simulink model "Racing_2019"  (R2017a)
settings: Solver=FixedStepDiscrete  StartTime=0.0  StopTime=Inf  FixedStep=1e-3  RelTol=1e-3  EnableMultiTasking=on
PostLoadFcn:
  | , if any(exist('dsrtsu_mdlpostloadfcn', 'file') == [2, 3, 6]), try dsrtsu_mdlpostloadfcn('Execute', bdroot); catch fprintf('Error in PostLoadFcn (dsrtsu_mdlpostloadfcn) for model "%s":\n %s\n', bdroot, lasterr); end, end,
undefined symbols (not defined in the file): Accu_Fans_Enable, Accu_Fans_ON, Accu_Fans_PWM, APPS_Bypass, APPS_Value, AUX_Error_Time, Batt_Temp_High_Threshold, Batt_Temp_Low_Threshold, BMS_Error_Time, BMS_Reset, BMS_Reset_Enable, BMS_Status_Bypass, Brake_Plausibility_Threshold, Brake_Threshold, Brakelight_Test, Braking_Torque, BSPD_State_Bypass, Buzzer, Buzzer_Silent, Buzzer_Test, Calibrate, CAN_Rx_FMEA_Enable, CAN_Status_FMEA_Enable, CAN_Tx_FMEA_Enable, Car_Reset, Car_Reset_Enable, Dash_Fan_PWM, DiscIntNeverNeededParam, DRS_Enable, DRS_PWM_OFF, DRS_PWM_ON, ED_Enable, ED_On, Eject_USB, Enable_Kill, Enable_LED_Test, Fans_Left_Enable, Fans_Left_ON, Fans_Left_PWM, Fans_Right_Enable, Fans_Right_ON, Fans_Right_PWM, I_MAX, IGBT_Temp_High_Threshold, IGBT_Temp_Low_Threshold, Inverter_CAN_Tx_Enable, Inverter_Frequency, KW_Max_Regen_Reset, KW_Max_Reset, LV_DCDC_Temp_High_Threshold, LV_DCDC_Temp_Low_Threshold, magnitude, Plausibility_Bypass, Power_Limiter_Killswitch, Power_Target_kW, Pump_Left_Enable, Pump_Left_ON, Pump_Right_Enable, Pump_Right_ON, Pump_Signal_Left ... (+13)
libraries: rtiusbflightreclib x206, simulink x153, rtican x52, powerlib_meascontrol x47, simulink_extras x17, rti1401lib_adc_type4 x6, rti1401lib_dio_type4 x3, rti1401lib_II_base x1
(part 19 of 23)

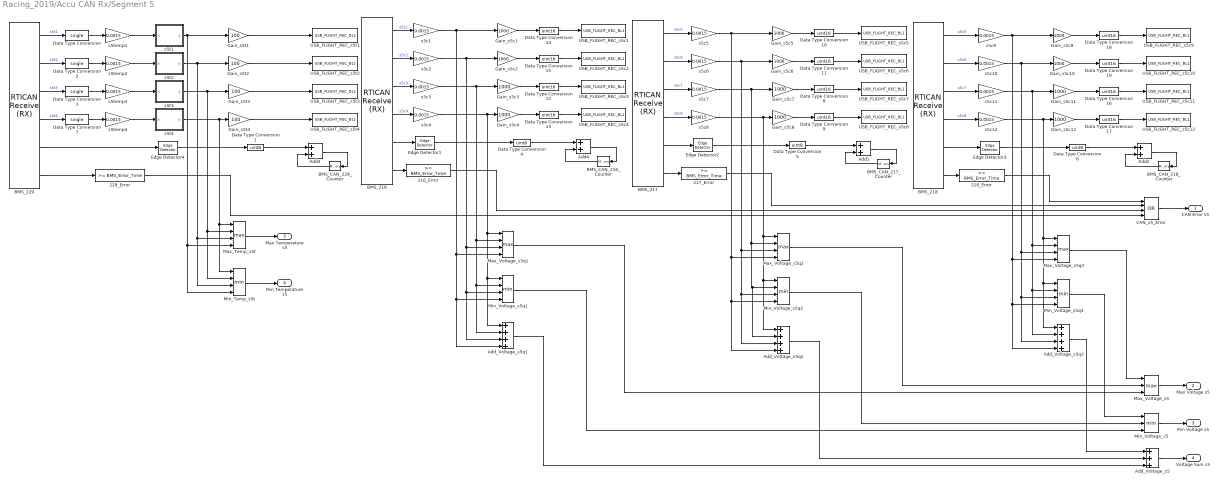
== system Racing_2019/Accu CAN Rx/Segment 5 ==
  216_Error : simulink/Logic and Bit Operations/Compare To Constant  relop=>=  const=BMS_Error_Time  OutDataTypeStr=boolean
  217_Error : simulink/Logic and Bit Operations/Compare To Constant  relop=>=  const=BMS_Error_Time  OutDataTypeStr=boolean
  218_Error : simulink/Logic and Bit Operations/Compare To Constant  relop=>=  const=BMS_Error_Time  OutDataTypeStr=boolean
  229_Error : simulink/Logic and Bit Operations/Compare To Constant  relop=>=  const=BMS_Error_Time  OutDataTypeStr=boolean
  Add{1..4} (4 alike) : Sum
  Add_Voltage_s5 : Sum  Inputs=+++
  Add_Voltage_s5q1 : Sum  Inputs=++++
  Add_Voltage_s5q2 : Sum  Inputs=++++
  Add_Voltage_s5q3 : Sum  Inputs=++++
  BMS_216 : rtican/RTICAN Receive (RX)   Reserved1=[]  Reserved2=[]  Reserved3=[]  Reserved4=[]  SfcnMessage=[]  Msg_Struct=[]  BoardTypeNo=[]  BoardNo=[]  ChannelNo=[]  Parameters=[]  DialogFcn=[]  UnitName=[]  Revision=[]  UnitValues=[]  DSProperties=struct('RTI',struct('Version',uint32(5),'BlockType',struct('isSLSource',uint8(1),'isSLSink',uint8(1),'isHWSource',uint8(0),'isHWSink',uint8(0),'isSetup',uint8(0),'isInline',uint8(1),'isNonInline',uint8(0),'isInterrupt',uint8(0),'isChannelwise',uint8(0)),'IOBoardType','RTICAN','UnitType','MESSAGE','Identifier','RX','DialogType','MSVC','BlockSet','RTICAN','SlaveProcessor','CAN'))  RTIBlockInterface=struct('OutputPortsWidth',int32([1 1 1 1 1 1]),'OutputPortsActive',[1 1 1 1 1 1],'OutputPortsName',{{'s5c1','s5c2','s5c3','s5c4',['RX status'],['RX delta time']}},'OutputPortsDataType',{{'SS_DOUBLE','SS_DOUBLE','SS_DOUBLE','SS_DOUBLE','SS_DOUBLE','SS_DOUBLE'}},'OutputPortsLabel',{{'s5c1','s5c2','s5c3','s5c4','',''}},'OutputPortsLabelMode','ON','InputPortsWidth',int32(0),'InputPortsActive',0,'DialogFcn','rtican_message_interface_gui','BlockDisplay',{{'','center'}},'IconTransparency','on','ParameterTunableNames',{{}},'InitLevel',3,'BlockName',struct('Token',{{'CAN_TYPE','_RX_M','_C'}},'BlockParam',{{'BoardTypeNo','BoardNo','ChannelNo'}}),'SampleTime',{{0.2}},'TriggerPort',{{'none'}},'EnablePort',{{'none'}})  RTIBlockParameters=struct('BoardTypeNo',{{1,'OFF',[]}},'BoardNo',{{2,'ON',[1 16]}},'ChannelNo',{{1,'ON',[1 2]}},'Parameters',{{struct('DataFileSupport',struct('DataFileSelectedMaster',0,'DataFileSelectedLocal',0,'DataFileName',['<no datafile support>|'],'DataFileDate','','SelectedFile',['<no file selected>']),'Options',struct('StatusSelected',1,'TimeSelected',0,'DeltaTimeSelected',1,'BytePortSelected',0,'MessageLengthSelected',0,'TriggerPort',struct('Selected',0,'TriggerType',0),'UserCoding',struct('Selected',0,'InterfaceFile','UserDecodingFile','FcnName','UserDecodeFcn','InportSelected',0,'InportWidth',1,'OutportSelected',0,'OutportWidth',1),'EnablePortSelected',0,'SignalOnPortnameSelected',1,'UseRXService',0),'Message',struct('MsgOnBlocknameSelected',0,'MsgName','BMS_s5q1','MsgIdFormat',0,'MsgId',216,'MsgLength',8,'NumSignals',4,'SampleTime',0.2,'Signal',struct('SgnName',{'s5c1','s5c2','s5c3','s5c4'},'SgnStartBit',{0,16,32,48},'SgnLength',{16,16,16,16},'SgnType',{0,0,0,0},'ModeValue',{-1,-1,-1,-1},'DataType',{0,0,0,0},'ByteLayout',{1,1,1,1},'Factor',{1,1,1,1},'Offset',{0,0,0,0},'SgnComment',{{''},{''},{''},{''}},'SgnUnit',{'','','',''},'Min',{0,0,0,0},'Max',{255,255,255,255},'SLDataType',{'SS_DOUBLE','SS_DOUBLE','SS_DOUBLE','SS_DOUBLE'}),'MsgIdNumFormat',0,'MsgComment',{{''}}),'Version',1.2,'general',struct('isFromLib',0)),'OFF',[]}},'GroupId',{{struct('Group',{{'RTICAN'}},'No',3,'Behavior',{{'NAMECHANGE'}},'BlockType',{{'SINK'}},'NameChangeFlag',0),'OFF',[]}},'SFcnRTICANMessage',{{struct('MsgType','RX','SFcnPortType','Scalar','MsgName','BMS_s5q1','MsgIdFormat','STD','MsgId',216,'MsgLength',8,'NumSignals',4,'SampleTime',0.2,'Signal',struct('SgnName',{'s5c1','s5c2','s5c3','s5c4'},'SgnStartBit',{0,16,32,48},'SgnLength',{16,16,16,16},'SgnType',{'standard','standard','standard','standard'},'ModeValue',{-1,-1,-1,-1},'DataType',{['unsigned int'],['unsigned int'],['unsigned int'],['unsigned int']},'ByteLayout',{['big endian'],['big endian'],['big endian'],['big endian']},'Factor',{1,1,1,1},'Offset',{0,0,0,0},'SLDataType',{'SS_DOUBLE','SS_DOUBLE','SS_DOUBLE','SS_DOUBLE'}),'StatusSelected','yes','TimeSelected','no','DeltaTimeSelected','yes','BytePortSelected','no','MessageLengthSelected','no','TriggerPort',struct('Selected','no','TriggerType',0),'UserCoding',struct('Selected','no','InterfaceFile','UserDecodingFile','FcnName','UserDecodeFcn','InportSelected','no','InportWidth',1,'OutportSelected','no','OutportWidth',1),'EnablePortSelected','no','UseRXService','no','BoardType','DS1','BoardNo',2,'ControllerNo',1),'OFF',[]}},'TLCFileName',{{'rtican_rx_message','OFF',[]}})  RTISFcnParameters=struct('SFcnRTICANMessage','struct','TLCFileName','char')  RTIBlockParaDefault=struct('BoardTypeNo',4302,'BoardNo',1,'ChannelNo',1,'Parameters',struct('DataFileSupport',struct('DataFileSelectedMaster',0,'DataFileSelectedLocal',0,'DataFileName','','DataFileDate','','SelectedFile',['<no file selected>']),'Options',struct('StatusSelected',1,'TimeSelected',1,'DeltaTimeSelected',1,'BytePortSelected',0,'MessageLengthSelected',0,'TriggerPort',struct('Selected',0,'TriggerType','rising'),'UserCoding',struct('Selected',0,'InterfaceFile','UserDecodingFile','FcnName','UserDecodeFcn','InportSelected',0,'InportWidth',1,'OutportSelected',0,'OutportWidth',1),'EnablePortSelected',0,'SignalOnPortnameSelected',1,'UseRXService',0),'Message',struct('MsgOnBlocknameSelected',0,'MsgName',['RX Message'],'MsgIdFormat',0,'MsgId',100,'MsgLength',8,'NumSignals',1,'SampleTime',-1,'Signal',struct('SgnName',['RX signal'],'SgnStartBit',0,'SgnLength',8,'SgnType',0,'ModeValue',-1,'DataType',0,'SLDataType','SS_DOUBLE','ByteLayout',0,'Factor',1,'Offset',0,'Min',0,'Max',255,'SgnComment',{{}},'SgnUnit',''),'MsgIdNumFormat',0,'MsgComment',{{''}}),'Version',1.2,'general',struct('isFromLib',1)),'GroupId',struct('Group',{{'RTICAN'}},'No',1,'Behavior',{{'NAMECHANGE'}},'BlockType',{{'SINK'}},'NameChangeFlag',0),'SFcnRTICANMessage',struct('MsgType','RX','MsgName',['RX Message'],'MsgIdFormat','STD','MsgId',100,'MsgLength',8,'NumSignals',1,'SampleTime',-1,'Signal',struct('SgnName',['RX signal'],'SgnStartBit',0,'SgnLength',8,'SgnType','standard','ModeValue',-1,'DataType',['unsigned int'],'ByteLayout',['little endian'],'SLDataType','SS_DOUBLE','Factor',1,'Offset',0),'StatusSelected','yes','TimeSelected','yes','DeltaTimeSelected','yes','BytePortSelected','no','MessageLengthSelected','no','EnablePortSelected','no','UserCoding',struct('Selected','no','InterfaceFile','UserDecodingFile','FcnName','UserDecodeFcn','InportSelected','no','InportWidth',1,'OutportSelected','no','OutportWidth',1),'TriggerPort',struct('Selected','no','TriggerType','rising'),'UseRXService','no','BoardType','DS4302','BoardNo',1,'ControllerNo',1,'SFcnPortType','Scalar'),'TLCFileName','rtican_rx_message')
      settings: AttributesFormatString=Group Id: RTICAN3\n  SourceProductName=dSPACE RTI CAN Blockset
  BMS_217 : rtican/RTICAN Receive (RX)   Reserved1=[]  Reserved2=[]  Reserved3=[]  Reserved4=[]  SfcnMessage=[]  Msg_Struct=[]  BoardTypeNo=[]  BoardNo=[]  ChannelNo=[]  Parameters=[]  DialogFcn=[]  UnitName=[]  Revision=[]  UnitValues=[]  DSProperties=struct('RTI',struct('Version',uint32(5),'BlockType',struct('isSLSource',uint8(1),'isSLSink',uint8(1),'isHWSource',uint8(0),'isHWSink',uint8(0),'isSetup',uint8(0),'isInline',uint8(1),'isNonInline',uint8(0),'isInterrupt',uint8(0),'isChannelwise',uint8(0)),'IOBoardType','RTICAN','UnitType','MESSAGE','Identifier','RX','DialogType','MSVC','BlockSet','RTICAN','SlaveProcessor','CAN'))  RTIBlockInterface=struct('OutputPortsWidth',int32([1 1 1 1 1 1]),'OutputPortsActive',[1 1 1 1 1 1],'OutputPortsName',{{'s5c5','s5c6','s5c7','s5c8',['RX status'],['RX delta time']}},'OutputPortsDataType',{{'SS_DOUBLE','SS_DOUBLE','SS_DOUBLE','SS_DOUBLE','SS_DOUBLE','SS_DOUBLE'}},'OutputPortsLabel',{{'s5c5','s5c6','s5c7','s5c8','',''}},'OutputPortsLabelMode','ON','InputPortsWidth',int32(0),'InputPortsActive',0,'DialogFcn','rtican_message_interface_gui','BlockDisplay',{{'','center'}},'IconTransparency','on','ParameterTunableNames',{{}},'InitLevel',3,'BlockName',struct('Token',{{'CAN_TYPE','_RX_M','_C'}},'BlockParam',{{'BoardTypeNo','BoardNo','ChannelNo'}}),'SampleTime',{{0.2}},'TriggerPort',{{'none'}},'EnablePort',{{'none'}})  RTIBlockParameters=struct('BoardTypeNo',{{1,'OFF',[]}},'BoardNo',{{2,'ON',[1 16]}},'ChannelNo',{{1,'ON',[1 2]}},'Parameters',{{struct('DataFileSupport',struct('DataFileSelectedMaster',0,'DataFileSelectedLocal',0,'DataFileName',['<no datafile support>|'],'DataFileDate','','SelectedFile',['<no file selected>']),'Options',struct('StatusSelected',1,'TimeSelected',0,'DeltaTimeSelected',1,'BytePortSelected',0,'MessageLengthSelected',0,'TriggerPort',struct('Selected',0,'TriggerType',0),'UserCoding',struct('Selected',0,'InterfaceFile','UserDecodingFile','FcnName','UserDecodeFcn','InportSelected',0,'InportWidth',1,'OutportSelected',0,'OutportWidth',1),'EnablePortSelected',0,'SignalOnPortnameSelected',1,'UseRXService',0),'Message',struct('MsgOnBlocknameSelected',0,'MsgName','BMS_s5q2','MsgIdFormat',0,'MsgId',217,'MsgLength',8,'NumSignals',4,'SampleTime',0.2,'Signal',struct('SgnName',{'s5c5','s5c6','s5c7','s5c8'},'SgnStartBit',{0,16,32,48},'SgnLength',{16,16,16,16},'SgnType',{0,0,0,0},'ModeValue',{-1,-1,-1,-1},'DataType',{0,0,0,0},'ByteLayout',{1,1,1,1},'Factor',{1,1,1,1},'Offset',{0,0,0,0},'SgnComment',{{''},{''},{''},{''}},'SgnUnit',{'','','',''},'Min',{0,0,0,0},'Max',{255,255,255,255},'SLDataType',{'SS_DOUBLE','SS_DOUBLE','SS_DOUBLE','SS_DOUBLE'}),'MsgIdNumFormat',0,'MsgComment',{{''}}),'Version',1.2,'general',struct('isFromLib',0)),'OFF',[]}},'GroupId',{{struct('Group',{{'RTICAN'}},'No',3,'Behavior',{{'NAMECHANGE'}},'BlockType',{{'SINK'}},'NameChangeFlag',0),'OFF',[]}},'SFcnRTICANMessage',{{struct('MsgType','RX','SFcnPortType','Scalar','MsgName','BMS_s5q2','MsgIdFormat','STD','MsgId',217,'MsgLength',8,'NumSignals',4,'SampleTime',0.2,'Signal',struct('SgnName',{'s5c5','s5c6','s5c7','s5c8'},'SgnStartBit',{0,16,32,48},'SgnLength',{16,16,16,16},'SgnType',{'standard','standard','standard','standard'},'ModeValue',{-1,-1,-1,-1},'DataType',{['unsigned int'],['unsigned int'],['unsigned int'],['unsigned int']},'ByteLayout',{['big endian'],['big endian'],['big endian'],['big endian']},'Factor',{1,1,1,1},'Offset',{0,0,0,0},'SLDataType',{'SS_DOUBLE','SS_DOUBLE','SS_DOUBLE','SS_DOUBLE'}),'StatusSelected','yes','TimeSelected','no','DeltaTimeSelected','yes','BytePortSelected','no','MessageLengthSelected','no','TriggerPort',struct('Selected','no','TriggerType',0),'UserCoding',struct('Selected','no','InterfaceFile','UserDecodingFile','FcnName','UserDecodeFcn','InportSelected','no','InportWidth',1,'OutportSelected','no','OutportWidth',1),'EnablePortSelected','no','UseRXService','no','BoardType','DS1','BoardNo',2,'ControllerNo',1),'OFF',[]}},'TLCFileName',{{'rtican_rx_message','OFF',[]}})  RTISFcnParameters=struct('SFcnRTICANMessage','struct','TLCFileName','char')  RTIBlockParaDefault=struct('BoardTypeNo',4302,'BoardNo',1,'ChannelNo',1,'Parameters',struct('DataFileSupport',struct('DataFileSelectedMaster',0,'DataFileSelectedLocal',0,'DataFileName','','DataFileDate','','SelectedFile',['<no file selected>']),'Options',struct('StatusSelected',1,'TimeSelected',1,'DeltaTimeSelected',1,'BytePortSelected',0,'MessageLengthSelected',0,'TriggerPort',struct('Selected',0,'TriggerType','rising'),'UserCoding',struct('Selected',0,'InterfaceFile','UserDecodingFile','FcnName','UserDecodeFcn','InportSelected',0,'InportWidth',1,'OutportSelected',0,'OutportWidth',1),'EnablePortSelected',0,'SignalOnPortnameSelected',1,'UseRXService',0),'Message',struct('MsgOnBlocknameSelected',0,'MsgName',['RX Message'],'MsgIdFormat',0,'MsgId',100,'MsgLength',8,'NumSignals',1,'SampleTime',-1,'Signal',struct('SgnName',['RX signal'],'SgnStartBit',0,'SgnLength',8,'SgnType',0,'ModeValue',-1,'DataType',0,'SLDataType','SS_DOUBLE','ByteLayout',0,'Factor',1,'Offset',0,'Min',0,'Max',255,'SgnComment',{{}},'SgnUnit',''),'MsgIdNumFormat',0,'MsgComment',{{''}}),'Version',1.2,'general',struct('isFromLib',1)),'GroupId',struct('Group',{{'RTICAN'}},'No',1,'Behavior',{{'NAMECHANGE'}},'BlockType',{{'SINK'}},'NameChangeFlag',0),'SFcnRTICANMessage',struct('MsgType','RX','MsgName',['RX Message'],'MsgIdFormat','STD','MsgId',100,'MsgLength',8,'NumSignals',1,'SampleTime',-1,'Signal',struct('SgnName',['RX signal'],'SgnStartBit',0,'SgnLength',8,'SgnType','standard','ModeValue',-1,'DataType',['unsigned int'],'ByteLayout',['little endian'],'SLDataType','SS_DOUBLE','Factor',1,'Offset',0),'StatusSelected','yes','TimeSelected','yes','DeltaTimeSelected','yes','BytePortSelected','no','MessageLengthSelected','no','EnablePortSelected','no','UserCoding',struct('Selected','no','InterfaceFile','UserDecodingFile','FcnName','UserDecodeFcn','InportSelected','no','InportWidth',1,'OutportSelected','no','OutportWidth',1),'TriggerPort',struct('Selected','no','TriggerType','rising'),'UseRXService','no','BoardType','DS4302','BoardNo',1,'ControllerNo',1,'SFcnPortType','Scalar'),'TLCFileName','rtican_rx_message')
      settings: AttributesFormatString=Group Id: RTICAN3\n  SourceProductName=dSPACE RTI CAN Blockset
  BMS_218 : rtican/RTICAN Receive (RX)   Reserved1=[]  Reserved2=[]  Reserved3=[]  Reserved4=[]  SfcnMessage=[]  Msg_Struct=[]  BoardTypeNo=[]  BoardNo=[]  ChannelNo=[]  Parameters=[]  DialogFcn=[]  UnitName=[]  Revision=[]  UnitValues=[]  DSProperties=struct('RTI',struct('Version',uint32(5),'BlockType',struct('isSLSource',uint8(1),'isSLSink',uint8(1),'isHWSource',uint8(0),'isHWSink',uint8(0),'isSetup',uint8(0),'isInline',uint8(1),'isNonInline',uint8(0),'isInterrupt',uint8(0),'isChannelwise',uint8(0)),'IOBoardType','RTICAN','UnitType','MESSAGE','Identifier','RX','DialogType','MSVC','BlockSet','RTICAN','SlaveProcessor','CAN'))  RTIBlockInterface=struct('OutputPortsWidth',int32([1 1 1 1 1 1]),'OutputPortsActive',[1 1 1 1 1 1],'OutputPortsName',{{'s5c5','s5c6','s5c7','s5c8',['RX status'],['RX delta time']}},'OutputPortsDataType',{{'SS_DOUBLE','SS_DOUBLE','SS_DOUBLE','SS_DOUBLE','SS_DOUBLE','SS_DOUBLE'}},'OutputPortsLabel',{{'s5c5','s5c6','s5c7','s5c8','',''}},'OutputPortsLabelMode','ON','InputPortsWidth',int32(0),'InputPortsActive',0,'DialogFcn','rtican_message_interface_gui','BlockDisplay',{{'','center'}},'IconTransparency','on','ParameterTunableNames',{{}},'InitLevel',3,'BlockName',struct('Token',{{'CAN_TYPE','_RX_M','_C'}},'BlockParam',{{'BoardTypeNo','BoardNo','ChannelNo'}}),'SampleTime',{{0.2}},'TriggerPort',{{'none'}},'EnablePort',{{'none'}})  RTIBlockParameters=struct('BoardTypeNo',{{1,'OFF',[]}},'BoardNo',{{2,'ON',[1 16]}},'ChannelNo',{{1,'ON',[1 2]}},'Parameters',{{struct('DataFileSupport',struct('DataFileSelectedMaster',0,'DataFileSelectedLocal',0,'DataFileName',['<no datafile support>|'],'DataFileDate','','SelectedFile',['<no file selected>']),'Options',struct('StatusSelected',1,'TimeSelected',0,'DeltaTimeSelected',1,'BytePortSelected',0,'MessageLengthSelected',0,'TriggerPort',struct('Selected',0,'TriggerType',0),'UserCoding',struct('Selected',0,'InterfaceFile','UserDecodingFile','FcnName','UserDecodeFcn','InportSelected',0,'InportWidth',1,'OutportSelected',0,'OutportWidth',1),'EnablePortSelected',0,'SignalOnPortnameSelected',1,'UseRXService',0),'Message',struct('MsgOnBlocknameSelected',0,'MsgName','BMS_s5q3','MsgIdFormat',0,'MsgId',218,'MsgLength',8,'NumSignals',4,'SampleTime',0.2,'Signal',struct('SgnName',{'s5c5','s5c6','s5c7','s5c8'},'SgnStartBit',{0,16,32,48},'SgnLength',{16,16,16,16},'SgnType',{0,0,0,0},'ModeValue',{-1,-1,-1,-1},'DataType',{0,0,0,0},'ByteLayout',{1,1,1,1},'Factor',{1,1,1,1},'Offset',{0,0,0,0},'SgnComment',{{''},{''},{''},{''}},'SgnUnit',{'','','',''},'Min',{0,0,0,0},'Max',{255,255,255,255},'SLDataType',{'SS_DOUBLE','SS_DOUBLE','SS_DOUBLE','SS_DOUBLE'}),'MsgIdNumFormat',0,'MsgComment',{{''}}),'Version',1.2,'general',struct('isFromLib',0)),'OFF',[]}},'GroupId',{{struct('Group',{{'RTICAN'}},'No',3,'Behavior',{{'NAMECHANGE'}},'BlockType',{{'SINK'}},'NameChangeFlag',0),'OFF',[]}},'SFcnRTICANMessage',{{struct('MsgType','RX','SFcnPortType','Scalar','MsgName','BMS_s5q3','MsgIdFormat','STD','MsgId',218,'MsgLength',8,'NumSignals',4,'SampleTime',0.2,'Signal',struct('SgnName',{'s5c5','s5c6','s5c7','s5c8'},'SgnStartBit',{0,16,32,48},'SgnLength',{16,16,16,16},'SgnType',{'standard','standard','standard','standard'},'ModeValue',{-1,-1,-1,-1},'DataType',{['unsigned int'],['unsigned int'],['unsigned int'],['unsigned int']},'ByteLayout',{['big endian'],['big endian'],['big endian'],['big endian']},'Factor',{1,1,1,1},'Offset',{0,0,0,0},'SLDataType',{'SS_DOUBLE','SS_DOUBLE','SS_DOUBLE','SS_DOUBLE'}),'StatusSelected','yes','TimeSelected','no','DeltaTimeSelected','yes','BytePortSelected','no','MessageLengthSelected','no','TriggerPort',struct('Selected','no','TriggerType',0),'UserCoding',struct('Selected','no','InterfaceFile','UserDecodingFile','FcnName','UserDecodeFcn','InportSelected','no','InportWidth',1,'OutportSelected','no','OutportWidth',1),'EnablePortSelected','no','UseRXService','no','BoardType','DS1','BoardNo',2,'ControllerNo',1),'OFF',[]}},'TLCFileName',{{'rtican_rx_message','OFF',[]}})  RTISFcnParameters=struct('SFcnRTICANMessage','struct','TLCFileName','char')  RTIBlockParaDefault=struct('BoardTypeNo',4302,'BoardNo',1,'ChannelNo',1,'Parameters',struct('DataFileSupport',struct('DataFileSelectedMaster',0,'DataFileSelectedLocal',0,'DataFileName','','DataFileDate','','SelectedFile',['<no file selected>']),'Options',struct('StatusSelected',1,'TimeSelected',1,'DeltaTimeSelected',1,'BytePortSelected',0,'MessageLengthSelected',0,'TriggerPort',struct('Selected',0,'TriggerType','rising'),'UserCoding',struct('Selected',0,'InterfaceFile','UserDecodingFile','FcnName','UserDecodeFcn','InportSelected',0,'InportWidth',1,'OutportSelected',0,'OutportWidth',1),'EnablePortSelected',0,'SignalOnPortnameSelected',1,'UseRXService',0),'Message',struct('MsgOnBlocknameSelected',0,'MsgName',['RX Message'],'MsgIdFormat',0,'MsgId',100,'MsgLength',8,'NumSignals',1,'SampleTime',-1,'Signal',struct('SgnName',['RX signal'],'SgnStartBit',0,'SgnLength',8,'SgnType',0,'ModeValue',-1,'DataType',0,'SLDataType','SS_DOUBLE','ByteLayout',0,'Factor',1,'Offset',0,'Min',0,'Max',255,'SgnComment',{{}},'SgnUnit',''),'MsgIdNumFormat',0,'MsgComment',{{''}}),'Version',1.2,'general',struct('isFromLib',1)),'GroupId',struct('Group',{{'RTICAN'}},'No',1,'Behavior',{{'NAMECHANGE'}},'BlockType',{{'SINK'}},'NameChangeFlag',0),'SFcnRTICANMessage',struct('MsgType','RX','MsgName',['RX Message'],'MsgIdFormat','STD','MsgId',100,'MsgLength',8,'NumSignals',1,'SampleTime',-1,'Signal',struct('SgnName',['RX signal'],'SgnStartBit',0,'SgnLength',8,'SgnType','standard','ModeValue',-1,'DataType',['unsigned int'],'ByteLayout',['little endian'],'SLDataType','SS_DOUBLE','Factor',1,'Offset',0),'StatusSelected','yes','TimeSelected','yes','DeltaTimeSelected','yes','BytePortSelected','no','MessageLengthSelected','no','EnablePortSelected','no','UserCoding',struct('Selected','no','InterfaceFile','UserDecodingFile','FcnName','UserDecodeFcn','InportSelected','no','InportWidth',1,'OutportSelected','no','OutportWidth',1),'TriggerPort',struct('Selected','no','TriggerType','rising'),'UseRXService','no','BoardType','DS4302','BoardNo',1,'ControllerNo',1,'SFcnPortType','Scalar'),'TLCFileName','rtican_rx_message')
      settings: AttributesFormatString=Group Id: RTICAN3\n  SourceProductName=dSPACE RTI CAN Blockset
  BMS_229 : rtican/RTICAN Receive (RX)   Reserved1=[]  Reserved2=[]  Reserved3=[]  Reserved4=[]  SfcnMessage=[]  Msg_Struct=[]  BoardTypeNo=[]  BoardNo=[]  ChannelNo=[]  Parameters=[]  DialogFcn=[]  UnitName=[]  Revision=[]  UnitValues=[]  DSProperties=struct('RTI',struct('Version',uint32(5),'BlockType',struct('isSLSource',uint8(1),'isSLSink',uint8(1),'isHWSource',uint8(0),'isHWSink',uint8(0),'isSetup',uint8(0),'isInline',uint8(1),'isNonInline',uint8(0),'isInterrupt',uint8(0),'isChannelwise',uint8(0)),'IOBoardType','RTICAN','UnitType','MESSAGE','Identifier','RX','DialogType','MSVC','BlockSet','RTICAN','SlaveProcessor','CAN'))  RTIBlockInterface=struct('OutputPortsWidth',int32([1 1 1 1 1 1]),'OutputPortsActive',[1 1 1 1 1 1],'OutputPortsName',{{'s5t1','s5t2','s5t3','s5t4',['RX status'],['RX delta time']}},'OutputPortsDataType',{{'SS_DOUBLE','SS_DOUBLE','SS_DOUBLE','SS_DOUBLE','SS_DOUBLE','SS_DOUBLE'}},'OutputPortsLabel',{{'s5t1','s5t2','s5t3','s5t4','',''}},'OutputPortsLabelMode','ON','InputPortsWidth',int32(0),'InputPortsActive',0,'DialogFcn','rtican_message_interface_gui','BlockDisplay',{{'','center'}},'IconTransparency','on','ParameterTunableNames',{{}},'InitLevel',3,'BlockName',struct('Token',{{'CAN_TYPE','_RX_M','_C'}},'BlockParam',{{'BoardTypeNo','BoardNo','ChannelNo'}}),'SampleTime',{{0.2}},'TriggerPort',{{'none'}},'EnablePort',{{'none'}})  RTIBlockParameters=struct('BoardTypeNo',{{1,'OFF',[]}},'BoardNo',{{2,'ON',[1 16]}},'ChannelNo',{{1,'ON',[1 2]}},'Parameters',{{struct('DataFileSupport',struct('DataFileSelectedMaster',0,'DataFileSelectedLocal',0,'DataFileName',['<no datafile support>|'],'DataFileDate','','SelectedFile',['<no file selected>']),'Options',struct('StatusSelected',1,'TimeSelected',0,'DeltaTimeSelected',1,'BytePortSelected',0,'MessageLengthSelected',0,'TriggerPort',struct('Selected',0,'TriggerType',0),'UserCoding',struct('Selected',0,'InterfaceFile','UserDecodingFile','FcnName','UserDecodeFcn','InportSelected',0,'InportWidth',1,'OutportSelected',0,'OutportWidth',1),'EnablePortSelected',0,'SignalOnPortnameSelected',1,'UseRXService',0),'Message',struct('MsgOnBlocknameSelected',0,'MsgName','BMS_s5t','MsgIdFormat',0,'MsgId',229,'MsgLength',8,'NumSignals',4,'SampleTime',0.2,'Signal',struct('SgnName',{'s5t1','s5t2','s5t3','s5t4'},'SgnStartBit',{0,16,32,48},'SgnLength',{16,16,16,16},'SgnType',{0,0,0,0},'ModeValue',{-1,-1,-1,-1},'DataType',{0,0,0,0},'ByteLayout',{1,1,1,1},'Factor',{1,1,1,1},'Offset',{0,0,0,0},'SgnComment',{{''},{''},{''},{''}},'SgnUnit',{'','','',''},'Min',{0,0,0,0},'Max',{255,255,255,255},'SLDataType',{'SS_DOUBLE','SS_DOUBLE','SS_DOUBLE','SS_DOUBLE'}),'MsgIdNumFormat',0,'MsgComment',{{''}}),'Version',1.2,'general',struct('isFromLib',0)),'OFF',[]}},'GroupId',{{struct('Group',{{'RTICAN'}},'No',3,'Behavior',{{'NAMECHANGE'}},'BlockType',{{'SINK'}},'NameChangeFlag',0),'OFF',[]}},'SFcnRTICANMessage',{{struct('MsgType','RX','SFcnPortType','Scalar','MsgName','BMS_s5t','MsgIdFormat','STD','MsgId',229,'MsgLength',8,'NumSignals',4,'SampleTime',0.2,'Signal',struct('SgnName',{'s5t1','s5t2','s5t3','s5t4'},'SgnStartBit',{0,16,32,48},'SgnLength',{16,16,16,16},'SgnType',{'standard','standard','standard','standard'},'ModeValue',{-1,-1,-1,-1},'DataType',{['unsigned int'],['unsigned int'],['unsigned int'],['unsigned int']},'ByteLayout',{['big endian'],['big endian'],['big endian'],['big endian']},'Factor',{1,1,1,1},'Offset',{0,0,0,0},'SLDataType',{'SS_DOUBLE','SS_DOUBLE','SS_DOUBLE','SS_DOUBLE'}),'StatusSelected','yes','TimeSelected','no','DeltaTimeSelected','yes','BytePortSelected','no','MessageLengthSelected','no','TriggerPort',struct('Selected','no','TriggerType',0),'UserCoding',struct('Selected','no','InterfaceFile','UserDecodingFile','FcnName','UserDecodeFcn','InportSelected','no','InportWidth',1,'OutportSelected','no','OutportWidth',1),'EnablePortSelected','no','UseRXService','no','BoardType','DS1','BoardNo',2,'ControllerNo',1),'OFF',[]}},'TLCFileName',{{'rtican_rx_message','OFF',[]}})  RTISFcnParameters=struct('SFcnRTICANMessage','struct','TLCFileName','char')  RTIBlockParaDefault=struct('BoardTypeNo',4302,'BoardNo',1,'ChannelNo',1,'Parameters',struct('DataFileSupport',struct('DataFileSelectedMaster',0,'DataFileSelectedLocal',0,'DataFileName','','DataFileDate','','SelectedFile',['<no file selected>']),'Options',struct('StatusSelected',1,'TimeSelected',1,'DeltaTimeSelected',1,'BytePortSelected',0,'MessageLengthSelected',0,'TriggerPort',struct('Selected',0,'TriggerType','rising'),'UserCoding',struct('Selected',0,'InterfaceFile','UserDecodingFile','FcnName','UserDecodeFcn','InportSelected',0,'InportWidth',1,'OutportSelected',0,'OutportWidth',1),'EnablePortSelected',0,'SignalOnPortnameSelected',1,'UseRXService',0),'Message',struct('MsgOnBlocknameSelected',0,'MsgName',['RX Message'],'MsgIdFormat',0,'MsgId',100,'MsgLength',8,'NumSignals',1,'SampleTime',-1,'Signal',struct('SgnName',['RX signal'],'SgnStartBit',0,'SgnLength',8,'SgnType',0,'ModeValue',-1,'DataType',0,'SLDataType','SS_DOUBLE','ByteLayout',0,'Factor',1,'Offset',0,'Min',0,'Max',255,'SgnComment',{{}},'SgnUnit',''),'MsgIdNumFormat',0,'MsgComment',{{''}}),'Version',1.2,'general',struct('isFromLib',1)),'GroupId',struct('Group',{{'RTICAN'}},'No',1,'Behavior',{{'NAMECHANGE'}},'BlockType',{{'SINK'}},'NameChangeFlag',0),'SFcnRTICANMessage',struct('MsgType','RX','MsgName',['RX Message'],'MsgIdFormat','STD','MsgId',100,'MsgLength',8,'NumSignals',1,'SampleTime',-1,'Signal',struct('SgnName',['RX signal'],'SgnStartBit',0,'SgnLength',8,'SgnType','standard','ModeValue',-1,'DataType',['unsigned int'],'ByteLayout',['little endian'],'SLDataType','SS_DOUBLE','Factor',1,'Offset',0),'StatusSelected','yes','TimeSelected','yes','DeltaTimeSelected','yes','BytePortSelected','no','MessageLengthSelected','no','EnablePortSelected','no','UserCoding',struct('Selected','no','InterfaceFile','UserDecodingFile','FcnName','UserDecodeFcn','InportSelected','no','InportWidth',1,'OutportSelected','no','OutportWidth',1),'TriggerPort',struct('Selected','no','TriggerType','rising'),'UseRXService','no','BoardType','DS4302','BoardNo',1,'ControllerNo',1,'SFcnPortType','Scalar'),'TLCFileName','rtican_rx_message')
      settings: AttributesFormatString=Group Id: RTICAN3\n  SourceProductName=dSPACE RTI CAN Blockset
  BMS_CAN_216_Counter : Memory  InheritSampleTime=on
  BMS_CAN_217_Counter : Memory  InheritSampleTime=on
  BMS_CAN_218_Counter : Memory  InheritSampleTime=on
  BMS_CAN_229_Counter : Memory  InheritSampleTime=on
  CAN_s5_Error : Logic  Operator=OR  Inputs=4  AllPortsSameDT=off  OutDataTypeStr=boolean
  Data Type Conversion{,2..3,7} (4 alike) : DataTypeConversion  OutDataTypeStr=single
  Data Type Conversion{1,4..6} (4 alike) : DataTypeConversion  OutDataTypeStr=uint8
  Data Type Conversion{8..19} (12 alike) : DataTypeConversion  OutDataTypeStr=uint16
  Edge Detector{1..4} (4 alike) : powerlib_meascontrol/Logic/Edge Detector  model=Rising  ic=0  Ts=-1
      settings: SourceProductName=Simscape Power Systems  SourceProductBaseCode=PS
  Gain_s5c{1..12} (12 alike) : Gain  Gain=1000
  Gain_s5t{1..4} (4 alike) : Gain  Gain=100
  Max_Temp_s5t : MinMax  Function=max  Inputs=4
  Max_Voltage_s5 : MinMax  Function=max  Inputs=3
  Max_Voltage_s5q1 : MinMax  Function=max  Inputs=4
  Max_Voltage_s5q2 : MinMax  Function=max  Inputs=4
  Max_Voltage_s5q3 : MinMax  Function=max  Inputs=4
  Min_Temp_s5t : MinMax  Inputs=4
  Min_Voltage_s5 : MinMax  Inputs=3
  Min_Voltage_s5q1 : MinMax  Inputs=4
  Min_Voltage_s5q2 : MinMax  Inputs=4
  Min_Voltage_s5q3 : MinMax  Inputs=4
  USB_FLIGHT_REC_s5c1 : rtiusbflightreclib/USB_FLIGHT_REC_BL1  VarName=s5c1  DataType=UInt16  SampleTime=-1  TLCFileName=rtiusbflightrecwrite  Reserved1=[]  Reserved2=[]  Reserved3=[]  Reserved4=[]  DSProperties=struct('RTI',struct('Version',uint32(3),'BlockType',struct('isSLSource',uint8(0),'isSLSink',uint8(1),'isHWSource',uint8(0),'isHWSink',uint8(0),'isSetup',uint8(0),'isInline',uint8(1),'isNonInline',uint8(0),'isInterrupt',uint8(0),'isChannelwise',uint8(0)),'IOBoardType',{{'DSUSB','FLIGHTREC'}},'UnitType','FLIGHTREC','Identifier','WRITE','DialogType','SL','BlockSet','RTIUSBFLIGHTREC','SlaveProcessor','NONE'))  RTIBlockInterface=struct('InputPortsActive',1,'InputPortsWidth',int32(1),'InputPortsDataType',{{'SS_UINT16'}},'BlockDisplay',{{['Write to\nUSB Flight Recorder'],'center'}},'IconTransparency','off','InitLevel',3,'BlockName',struct('Token',{{'USB_FLIGHT_REC_BL1'}}),'MaskDescription',['Write input to the Flight Recorder. Recorded data can be referenced by the specified variable.'],'SampleTime',{{-1}})  RTIBlockParameters=struct('VarName',{{'s5c1','OFF',[]}},'DataType',{{'UInt16','OFF',[]}},'SampleTime',{{-1,'OFF',[]}},'TLCFileName',{{'rtiusbflightrecwrite','OFF',[]}})  RTISFcnParameters=struct('VarName','char','DataType','char','SampleTime','double','TLCFileName','char')  RTIBlockParaDefault=struct('VarName','Var1','DataType','Single','SampleTime',-1,'TLCFileName','rtiusbflightrecwrite')
      settings: SourceProductName=dSPACE RTI USB Flight Rec Blockset
  USB_FLIGHT_REC_s5c10 : rtiusbflightreclib/USB_FLIGHT_REC_BL1  VarName=s5c10  DataType=UInt16  SampleTime=-1  TLCFileName=rtiusbflightrecwrite  Reserved1=[]  Reserved2=[]  Reserved3=[]  Reserved4=[]  DSProperties=struct('RTI',struct('Version',uint32(3),'BlockType',struct('isSLSource',uint8(0),'isSLSink',uint8(1),'isHWSource',uint8(0),'isHWSink',uint8(0),'isSetup',uint8(0),'isInline',uint8(1),'isNonInline',uint8(0),'isInterrupt',uint8(0),'isChannelwise',uint8(0)),'IOBoardType',{{'DSUSB','FLIGHTREC'}},'UnitType','FLIGHTREC','Identifier','WRITE','DialogType','SL','BlockSet','RTIUSBFLIGHTREC','SlaveProcessor','NONE'))  RTIBlockInterface=struct('InputPortsActive',1,'InputPortsWidth',int32(1),'InputPortsDataType',{{'SS_UINT16'}},'BlockDisplay',{{['Write to\nUSB Flight Recorder'],'center'}},'IconTransparency','off','InitLevel',3,'BlockName',struct('Token',{{'USB_FLIGHT_REC_BL1'}}),'MaskDescription',['Write input to the Flight Recorder. Recorded data can be referenced by the specified variable.'],'SampleTime',{{-1}})  RTIBlockParameters=struct('VarName',{{'s5c10','OFF',[]}},'DataType',{{'UInt16','OFF',[]}},'SampleTime',{{-1,'OFF',[]}},'TLCFileName',{{'rtiusbflightrecwrite','OFF',[]}})  RTISFcnParameters=struct('VarName','char','DataType','char','SampleTime','double','TLCFileName','char')  RTIBlockParaDefault=struct('VarName','Var1','DataType','Single','SampleTime',-1,'TLCFileName','rtiusbflightrecwrite')
      settings: SourceProductName=dSPACE RTI USB Flight Rec Blockset
  USB_FLIGHT_REC_s5c11 : rtiusbflightreclib/USB_FLIGHT_REC_BL1  VarName=s5c11  DataType=UInt16  SampleTime=-1  TLCFileName=rtiusbflightrecwrite  Reserved1=[]  Reserved2=[]  Reserved3=[]  Reserved4=[]  DSProperties=struct('RTI',struct('Version',uint32(3),'BlockType',struct('isSLSource',uint8(0),'isSLSink',uint8(1),'isHWSource',uint8(0),'isHWSink',uint8(0),'isSetup',uint8(0),'isInline',uint8(1),'isNonInline',uint8(0),'isInterrupt',uint8(0),'isChannelwise',uint8(0)),'IOBoardType',{{'DSUSB','FLIGHTREC'}},'UnitType','FLIGHTREC','Identifier','WRITE','DialogType','SL','BlockSet','RTIUSBFLIGHTREC','SlaveProcessor','NONE'))  RTIBlockInterface=struct('InputPortsActive',1,'InputPortsWidth',int32(1),'InputPortsDataType',{{'SS_UINT16'}},'BlockDisplay',{{['Write to\nUSB Flight Recorder'],'center'}},'IconTransparency','off','InitLevel',3,'BlockName',struct('Token',{{'USB_FLIGHT_REC_BL1'}}),'MaskDescription',['Write input to the Flight Recorder. Recorded data can be referenced by the specified variable.'],'SampleTime',{{-1}})  RTIBlockParameters=struct('VarName',{{'s5c11','OFF',[]}},'DataType',{{'UInt16','OFF',[]}},'SampleTime',{{-1,'OFF',[]}},'TLCFileName',{{'rtiusbflightrecwrite','OFF',[]}})  RTISFcnParameters=struct('VarName','char','DataType','char','SampleTime','double','TLCFileName','char')  RTIBlockParaDefault=struct('VarName','Var1','DataType','Single','SampleTime',-1,'TLCFileName','rtiusbflightrecwrite')
      settings: SourceProductName=dSPACE RTI USB Flight Rec Blockset
  USB_FLIGHT_REC_s5c12 : rtiusbflightreclib/USB_FLIGHT_REC_BL1  VarName=s5c12  DataType=UInt16  SampleTime=-1  TLCFileName=rtiusbflightrecwrite  Reserved1=[]  Reserved2=[]  Reserved3=[]  Reserved4=[]  DSProperties=struct('RTI',struct('Version',uint32(3),'BlockType',struct('isSLSource',uint8(0),'isSLSink',uint8(1),'isHWSource',uint8(0),'isHWSink',uint8(0),'isSetup',uint8(0),'isInline',uint8(1),'isNonInline',uint8(0),'isInterrupt',uint8(0),'isChannelwise',uint8(0)),'IOBoardType',{{'DSUSB','FLIGHTREC'}},'UnitType','FLIGHTREC','Identifier','WRITE','DialogType','SL','BlockSet','RTIUSBFLIGHTREC','SlaveProcessor','NONE'))  RTIBlockInterface=struct('InputPortsActive',1,'InputPortsWidth',int32(1),'InputPortsDataType',{{'SS_UINT16'}},'BlockDisplay',{{['Write to\nUSB Flight Recorder'],'center'}},'IconTransparency','off','InitLevel',3,'BlockName',struct('Token',{{'USB_FLIGHT_REC_BL1'}}),'MaskDescription',['Write input to the Flight Recorder. Recorded data can be referenced by the specified variable.'],'SampleTime',{{-1}})  RTIBlockParameters=struct('VarName',{{'s5c12','OFF',[]}},'DataType',{{'UInt16','OFF',[]}},'SampleTime',{{-1,'OFF',[]}},'TLCFileName',{{'rtiusbflightrecwrite','OFF',[]}})  RTISFcnParameters=struct('VarName','char','DataType','char','SampleTime','double','TLCFileName','char')  RTIBlockParaDefault=struct('VarName','Var1','DataType','Single','SampleTime',-1,'TLCFileName','rtiusbflightrecwrite')
      settings: SourceProductName=dSPACE RTI USB Flight Rec Blockset
  USB_FLIGHT_REC_s5c2 : rtiusbflightreclib/USB_FLIGHT_REC_BL1  VarName=s5c2  DataType=UInt16  SampleTime=-1  TLCFileName=rtiusbflightrecwrite  Reserved1=[]  Reserved2=[]  Reserved3=[]  Reserved4=[]  DSProperties=struct('RTI',struct('Version',uint32(3),'BlockType',struct('isSLSource',uint8(0),'isSLSink',uint8(1),'isHWSource',uint8(0),'isHWSink',uint8(0),'isSetup',uint8(0),'isInline',uint8(1),'isNonInline',uint8(0),'isInterrupt',uint8(0),'isChannelwise',uint8(0)),'IOBoardType',{{'DSUSB','FLIGHTREC'}},'UnitType','FLIGHTREC','Identifier','WRITE','DialogType','SL','BlockSet','RTIUSBFLIGHTREC','SlaveProcessor','NONE'))  RTIBlockInterface=struct('InputPortsActive',1,'InputPortsWidth',int32(1),'InputPortsDataType',{{'SS_UINT16'}},'BlockDisplay',{{['Write to\nUSB Flight Recorder'],'center'}},'IconTransparency','off','InitLevel',3,'BlockName',struct('Token',{{'USB_FLIGHT_REC_BL1'}}),'MaskDescription',['Write input to the Flight Recorder. Recorded data can be referenced by the specified variable.'],'SampleTime',{{-1}})  RTIBlockParameters=struct('VarName',{{'s5c2','OFF',[]}},'DataType',{{'UInt16','OFF',[]}},'SampleTime',{{-1,'OFF',[]}},'TLCFileName',{{'rtiusbflightrecwrite','OFF',[]}})  RTISFcnParameters=struct('VarName','char','DataType','char','SampleTime','double','TLCFileName','char')  RTIBlockParaDefault=struct('VarName','Var1','DataType','Single','SampleTime',-1,'TLCFileName','rtiusbflightrecwrite')
      settings: SourceProductName=dSPACE RTI USB Flight Rec Blockset
  USB_FLIGHT_REC_s5c3 : rtiusbflightreclib/USB_FLIGHT_REC_BL1  VarName=s5c3  DataType=UInt16  SampleTime=-1  TLCFileName=rtiusbflightrecwrite  Reserved1=[]  Reserved2=[]  Reserved3=[]  Reserved4=[]  DSProperties=struct('RTI',struct('Version',uint32(3),'BlockType',struct('isSLSource',uint8(0),'isSLSink',uint8(1),'isHWSource',uint8(0),'isHWSink',uint8(0),'isSetup',uint8(0),'isInline',uint8(1),'isNonInline',uint8(0),'isInterrupt',uint8(0),'isChannelwise',uint8(0)),'IOBoardType',{{'DSUSB','FLIGHTREC'}},'UnitType','FLIGHTREC','Identifier','WRITE','DialogType','SL','BlockSet','RTIUSBFLIGHTREC','SlaveProcessor','NONE'))  RTIBlockInterface=struct('InputPortsActive',1,'InputPortsWidth',int32(1),'InputPortsDataType',{{'SS_UINT16'}},'BlockDisplay',{{['Write to\nUSB Flight Recorder'],'center'}},'IconTransparency','off','InitLevel',3,'BlockName',struct('Token',{{'USB_FLIGHT_REC_BL1'}}),'MaskDescription',['Write input to the Flight Recorder. Recorded data can be referenced by the specified variable.'],'SampleTime',{{-1}})  RTIBlockParameters=struct('VarName',{{'s5c3','OFF',[]}},'DataType',{{'UInt16','OFF',[]}},'SampleTime',{{-1,'OFF',[]}},'TLCFileName',{{'rtiusbflightrecwrite','OFF',[]}})  RTISFcnParameters=struct('VarName','char','DataType','char','SampleTime','double','TLCFileName','char')  RTIBlockParaDefault=struct('VarName','Var1','DataType','Single','SampleTime',-1,'TLCFileName','rtiusbflightrecwrite')
      settings: SourceProductName=dSPACE RTI USB Flight Rec Blockset
  USB_FLIGHT_REC_s5c4 : rtiusbflightreclib/USB_FLIGHT_REC_BL1  VarName=s5c4  DataType=UInt16  SampleTime=-1  TLCFileName=rtiusbflightrecwrite  Reserved1=[]  Reserved2=[]  Reserved3=[]  Reserved4=[]  DSProperties=struct('RTI',struct('Version',uint32(3),'BlockType',struct('isSLSource',uint8(0),'isSLSink',uint8(1),'isHWSource',uint8(0),'isHWSink',uint8(0),'isSetup',uint8(0),'isInline',uint8(1),'isNonInline',uint8(0),'isInterrupt',uint8(0),'isChannelwise',uint8(0)),'IOBoardType',{{'DSUSB','FLIGHTREC'}},'UnitType','FLIGHTREC','Identifier','WRITE','DialogType','SL','BlockSet','RTIUSBFLIGHTREC','SlaveProcessor','NONE'))  RTIBlockInterface=struct('InputPortsActive',1,'InputPortsWidth',int32(1),'InputPortsDataType',{{'SS_UINT16'}},'BlockDisplay',{{['Write to\nUSB Flight Recorder'],'center'}},'IconTransparency','off','InitLevel',3,'BlockName',struct('Token',{{'USB_FLIGHT_REC_BL1'}}),'MaskDescription',['Write input to the Flight Recorder. Recorded data can be referenced by the specified variable.'],'SampleTime',{{-1}})  RTIBlockParameters=struct('VarName',{{'s5c4','OFF',[]}},'DataType',{{'UInt16','OFF',[]}},'SampleTime',{{-1,'OFF',[]}},'TLCFileName',{{'rtiusbflightrecwrite','OFF',[]}})  RTISFcnParameters=struct('VarName','char','DataType','char','SampleTime','double','TLCFileName','char')  RTIBlockParaDefault=struct('VarName','Var1','DataType','Single','SampleTime',-1,'TLCFileName','rtiusbflightrecwrite')
      settings: SourceProductName=dSPACE RTI USB Flight Rec Blockset
  USB_FLIGHT_REC_s5c5 : rtiusbflightreclib/USB_FLIGHT_REC_BL1  VarName=s5c5  DataType=UInt16  SampleTime=-1  TLCFileName=rtiusbflightrecwrite  Reserved1=[]  Reserved2=[]  Reserved3=[]  Reserved4=[]  DSProperties=struct('RTI',struct('Version',uint32(3),'BlockType',struct('isSLSource',uint8(0),'isSLSink',uint8(1),'isHWSource',uint8(0),'isHWSink',uint8(0),'isSetup',uint8(0),'isInline',uint8(1),'isNonInline',uint8(0),'isInterrupt',uint8(0),'isChannelwise',uint8(0)),'IOBoardType',{{'DSUSB','FLIGHTREC'}},'UnitType','FLIGHTREC','Identifier','WRITE','DialogType','SL','BlockSet','RTIUSBFLIGHTREC','SlaveProcessor','NONE'))  RTIBlockInterface=struct('InputPortsActive',1,'InputPortsWidth',int32(1),'InputPortsDataType',{{'SS_UINT16'}},'BlockDisplay',{{['Write to\nUSB Flight Recorder'],'center'}},'IconTransparency','off','InitLevel',3,'BlockName',struct('Token',{{'USB_FLIGHT_REC_BL1'}}),'MaskDescription',['Write input to the Flight Recorder. Recorded data can be referenced by the specified variable.'],'SampleTime',{{-1}})  RTIBlockParameters=struct('VarName',{{'s5c5','OFF',[]}},'DataType',{{'UInt16','OFF',[]}},'SampleTime',{{-1,'OFF',[]}},'TLCFileName',{{'rtiusbflightrecwrite','OFF',[]}})  RTISFcnParameters=struct('VarName','char','DataType','char','SampleTime','double','TLCFileName','char')  RTIBlockParaDefault=struct('VarName','Var1','DataType','Single','SampleTime',-1,'TLCFileName','rtiusbflightrecwrite')
      settings: SourceProductName=dSPACE RTI USB Flight Rec Blockset
  USB_FLIGHT_REC_s5c6 : rtiusbflightreclib/USB_FLIGHT_REC_BL1  VarName=s5c6  DataType=UInt16  SampleTime=-1  TLCFileName=rtiusbflightrecwrite  Reserved1=[]  Reserved2=[]  Reserved3=[]  Reserved4=[]  DSProperties=struct('RTI',struct('Version',uint32(3),'BlockType',struct('isSLSource',uint8(0),'isSLSink',uint8(1),'isHWSource',uint8(0),'isHWSink',uint8(0),'isSetup',uint8(0),'isInline',uint8(1),'isNonInline',uint8(0),'isInterrupt',uint8(0),'isChannelwise',uint8(0)),'IOBoardType',{{'DSUSB','FLIGHTREC'}},'UnitType','FLIGHTREC','Identifier','WRITE','DialogType','SL','BlockSet','RTIUSBFLIGHTREC','SlaveProcessor','NONE'))  RTIBlockInterface=struct('InputPortsActive',1,'InputPortsWidth',int32(1),'InputPortsDataType',{{'SS_UINT16'}},'BlockDisplay',{{['Write to\nUSB Flight Recorder'],'center'}},'IconTransparency','off','InitLevel',3,'BlockName',struct('Token',{{'USB_FLIGHT_REC_BL1'}}),'MaskDescription',['Write input to the Flight Recorder. Recorded data can be referenced by the specified variable.'],'SampleTime',{{-1}})  RTIBlockParameters=struct('VarName',{{'s5c6','OFF',[]}},'DataType',{{'UInt16','OFF',[]}},'SampleTime',{{-1,'OFF',[]}},'TLCFileName',{{'rtiusbflightrecwrite','OFF',[]}})  RTISFcnParameters=struct('VarName','char','DataType','char','SampleTime','double','TLCFileName','char')  RTIBlockParaDefault=struct('VarName','Var1','DataType','Single','SampleTime',-1,'TLCFileName','rtiusbflightrecwrite')
      settings: SourceProductName=dSPACE RTI USB Flight Rec Blockset
  USB_FLIGHT_REC_s5c7 : rtiusbflightreclib/USB_FLIGHT_REC_BL1  VarName=s5c7  DataType=UInt16  SampleTime=-1  TLCFileName=rtiusbflightrecwrite  Reserved1=[]  Reserved2=[]  Reserved3=[]  Reserved4=[]  DSProperties=struct('RTI',struct('Version',uint32(3),'BlockType',struct('isSLSource',uint8(0),'isSLSink',uint8(1),'isHWSource',uint8(0),'isHWSink',uint8(0),'isSetup',uint8(0),'isInline',uint8(1),'isNonInline',uint8(0),'isInterrupt',uint8(0),'isChannelwise',uint8(0)),'IOBoardType',{{'DSUSB','FLIGHTREC'}},'UnitType','FLIGHTREC','Identifier','WRITE','DialogType','SL','BlockSet','RTIUSBFLIGHTREC','SlaveProcessor','NONE'))  RTIBlockInterface=struct('InputPortsActive',1,'InputPortsWidth',int32(1),'InputPortsDataType',{{'SS_UINT16'}},'BlockDisplay',{{['Write to\nUSB Flight Recorder'],'center'}},'IconTransparency','off','InitLevel',3,'BlockName',struct('Token',{{'USB_FLIGHT_REC_BL1'}}),'MaskDescription',['Write input to the Flight Recorder. Recorded data can be referenced by the specified variable.'],'SampleTime',{{-1}})  RTIBlockParameters=struct('VarName',{{'s5c7','OFF',[]}},'DataType',{{'UInt16','OFF',[]}},'SampleTime',{{-1,'OFF',[]}},'TLCFileName',{{'rtiusbflightrecwrite','OFF',[]}})  RTISFcnParameters=struct('VarName','char','DataType','char','SampleTime','double','TLCFileName','char')  RTIBlockParaDefault=struct('VarName','Var1','DataType','Single','SampleTime',-1,'TLCFileName','rtiusbflightrecwrite')
      settings: SourceProductName=dSPACE RTI USB Flight Rec Blockset
  USB_FLIGHT_REC_s5c8 : rtiusbflightreclib/USB_FLIGHT_REC_BL1  VarName=s5c8  DataType=UInt16  SampleTime=-1  TLCFileName=rtiusbflightrecwrite  Reserved1=[]  Reserved2=[]  Reserved3=[]  Reserved4=[]  DSProperties=struct('RTI',struct('Version',uint32(3),'BlockType',struct('isSLSource',uint8(0),'isSLSink',uint8(1),'isHWSource',uint8(0),'isHWSink',uint8(0),'isSetup',uint8(0),'isInline',uint8(1),'isNonInline',uint8(0),'isInterrupt',uint8(0),'isChannelwise',uint8(0)),'IOBoardType',{{'DSUSB','FLIGHTREC'}},'UnitType','FLIGHTREC','Identifier','WRITE','DialogType','SL','BlockSet','RTIUSBFLIGHTREC','SlaveProcessor','NONE'))  RTIBlockInterface=struct('InputPortsActive',1,'InputPortsWidth',int32(1),'InputPortsDataType',{{'SS_UINT16'}},'BlockDisplay',{{['Write to\nUSB Flight Recorder'],'center'}},'IconTransparency','off','InitLevel',3,'BlockName',struct('Token',{{'USB_FLIGHT_REC_BL1'}}),'MaskDescription',['Write input to the Flight Recorder. Recorded data can be referenced by the specified variable.'],'SampleTime',{{-1}})  RTIBlockParameters=struct('VarName',{{'s5c8','OFF',[]}},'DataType',{{'UInt16','OFF',[]}},'SampleTime',{{-1,'OFF',[]}},'TLCFileName',{{'rtiusbflightrecwrite','OFF',[]}})  RTISFcnParameters=struct('VarName','char','DataType','char','SampleTime','double','TLCFileName','char')  RTIBlockParaDefault=struct('VarName','Var1','DataType','Single','SampleTime',-1,'TLCFileName','rtiusbflightrecwrite')
      settings: SourceProductName=dSPACE RTI USB Flight Rec Blockset
  USB_FLIGHT_REC_s5c9 : rtiusbflightreclib/USB_FLIGHT_REC_BL1  VarName=s5c9  DataType=UInt16  SampleTime=-1  TLCFileName=rtiusbflightrecwrite  Reserved1=[]  Reserved2=[]  Reserved3=[]  Reserved4=[]  DSProperties=struct('RTI',struct('Version',uint32(3),'BlockType',struct('isSLSource',uint8(0),'isSLSink',uint8(1),'isHWSource',uint8(0),'isHWSink',uint8(0),'isSetup',uint8(0),'isInline',uint8(1),'isNonInline',uint8(0),'isInterrupt',uint8(0),'isChannelwise',uint8(0)),'IOBoardType',{{'DSUSB','FLIGHTREC'}},'UnitType','FLIGHTREC','Identifier','WRITE','DialogType','SL','BlockSet','RTIUSBFLIGHTREC','SlaveProcessor','NONE'))  RTIBlockInterface=struct('InputPortsActive',1,'InputPortsWidth',int32(1),'InputPortsDataType',{{'SS_UINT16'}},'BlockDisplay',{{['Write to\nUSB Flight Recorder'],'center'}},'IconTransparency','off','InitLevel',3,'BlockName',struct('Token',{{'USB_FLIGHT_REC_BL1'}}),'MaskDescription',['Write input to the Flight Recorder. Recorded data can be referenced by the specified variable.'],'SampleTime',{{-1}})  RTIBlockParameters=struct('VarName',{{'s5c9','OFF',[]}},'DataType',{{'UInt16','OFF',[]}},'SampleTime',{{-1,'OFF',[]}},'TLCFileName',{{'rtiusbflightrecwrite','OFF',[]}})  RTISFcnParameters=struct('VarName','char','DataType','char','SampleTime','double','TLCFileName','char')  RTIBlockParaDefault=struct('VarName','Var1','DataType','Single','SampleTime',-1,'TLCFileName','rtiusbflightrecwrite')
      settings: SourceProductName=dSPACE RTI USB Flight Rec Blockset
  USB_FLIGHT_REC_s5t1 : rtiusbflightreclib/USB_FLIGHT_REC_BL1  VarName=s5t1  DataType=Single  SampleTime=-1  TLCFileName=rtiusbflightrecwrite  Reserved1=[]  Reserved2=[]  Reserved3=[]  Reserved4=[]  DSProperties=struct('RTI',struct('Version',uint32(3),'BlockType',struct('isSLSource',uint8(0),'isSLSink',uint8(1),'isHWSource',uint8(0),'isHWSink',uint8(0),'isSetup',uint8(0),'isInline',uint8(1),'isNonInline',uint8(0),'isInterrupt',uint8(0),'isChannelwise',uint8(0)),'IOBoardType',{{'DSUSB','FLIGHTREC'}},'UnitType','FLIGHTREC','Identifier','WRITE','DialogType','SL','BlockSet','RTIUSBFLIGHTREC','SlaveProcessor','NONE'))  RTIBlockInterface=struct('InputPortsActive',1,'InputPortsWidth',int32(1),'InputPortsDataType',{{'SS_SINGLE'}},'BlockDisplay',{{['Write to\nUSB Flight Recorder'],'center'}},'IconTransparency','off','InitLevel',3,'BlockName',struct('Token',{{'USB_FLIGHT_REC_BL1'}}),'MaskDescription',['Write input to the Flight Recorder. Recorded data can be referenced by the specified variable.'],'SampleTime',{{-1}})  RTIBlockParameters=struct('VarName',{{'s5t1','OFF',[]}},'DataType',{{'Single','OFF',[]}},'SampleTime',{{-1,'OFF',[]}},'TLCFileName',{{'rtiusbflightrecwrite','OFF',[]}})  RTISFcnParameters=struct('VarName','char','DataType','char','SampleTime','double','TLCFileName','char')  RTIBlockParaDefault=struct('VarName','Var1','DataType','Single','SampleTime',-1,'TLCFileName','rtiusbflightrecwrite')
      settings: SourceProductName=dSPACE RTI USB Flight Rec Blockset
  USB_FLIGHT_REC_s5t2 : rtiusbflightreclib/USB_FLIGHT_REC_BL1  VarName=s5t2  DataType=Single  SampleTime=-1  TLCFileName=rtiusbflightrecwrite  Reserved1=[]  Reserved2=[]  Reserved3=[]  Reserved4=[]  DSProperties=struct('RTI',struct('Version',uint32(3),'BlockType',struct('isSLSource',uint8(0),'isSLSink',uint8(1),'isHWSource',uint8(0),'isHWSink',uint8(0),'isSetup',uint8(0),'isInline',uint8(1),'isNonInline',uint8(0),'isInterrupt',uint8(0),'isChannelwise',uint8(0)),'IOBoardType',{{'DSUSB','FLIGHTREC'}},'UnitType','FLIGHTREC','Identifier','WRITE','DialogType','SL','BlockSet','RTIUSBFLIGHTREC','SlaveProcessor','NONE'))  RTIBlockInterface=struct('InputPortsActive',1,'InputPortsWidth',int32(1),'InputPortsDataType',{{'SS_SINGLE'}},'BlockDisplay',{{['Write to\nUSB Flight Recorder'],'center'}},'IconTransparency','off','InitLevel',3,'BlockName',struct('Token',{{'USB_FLIGHT_REC_BL1'}}),'MaskDescription',['Write input to the Flight Recorder. Recorded data can be referenced by the specified variable.'],'SampleTime',{{-1}})  RTIBlockParameters=struct('VarName',{{'s5t2','OFF',[]}},'DataType',{{'Single','OFF',[]}},'SampleTime',{{-1,'OFF',[]}},'TLCFileName',{{'rtiusbflightrecwrite','OFF',[]}})  RTISFcnParameters=struct('VarName','char','DataType','char','SampleTime','double','TLCFileName','char')  RTIBlockParaDefault=struct('VarName','Var1','DataType','Single','SampleTime',-1,'TLCFileName','rtiusbflightrecwrite')
      settings: SourceProductName=dSPACE RTI USB Flight Rec Blockset
  USB_FLIGHT_REC_s5t3 : rtiusbflightreclib/USB_FLIGHT_REC_BL1  VarName=s5t3  DataType=Single  SampleTime=-1  TLCFileName=rtiusbflightrecwrite  Reserved1=[]  Reserved2=[]  Reserved3=[]  Reserved4=[]  DSProperties=struct('RTI',struct('Version',uint32(3),'BlockType',struct('isSLSource',uint8(0),'isSLSink',uint8(1),'isHWSource',uint8(0),'isHWSink',uint8(0),'isSetup',uint8(0),'isInline',uint8(1),'isNonInline',uint8(0),'isInterrupt',uint8(0),'isChannelwise',uint8(0)),'IOBoardType',{{'DSUSB','FLIGHTREC'}},'UnitType','FLIGHTREC','Identifier','WRITE','DialogType','SL','BlockSet','RTIUSBFLIGHTREC','SlaveProcessor','NONE'))  RTIBlockInterface=struct('InputPortsActive',1,'InputPortsWidth',int32(1),'InputPortsDataType',{{'SS_SINGLE'}},'BlockDisplay',{{['Write to\nUSB Flight Recorder'],'center'}},'IconTransparency','off','InitLevel',3,'BlockName',struct('Token',{{'USB_FLIGHT_REC_BL1'}}),'MaskDescription',['Write input to the Flight Recorder. Recorded data can be referenced by the specified variable.'],'SampleTime',{{-1}})  RTIBlockParameters=struct('VarName',{{'s5t3','OFF',[]}},'DataType',{{'Single','OFF',[]}},'SampleTime',{{-1,'OFF',[]}},'TLCFileName',{{'rtiusbflightrecwrite','OFF',[]}})  RTISFcnParameters=struct('VarName','char','DataType','char','SampleTime','double','TLCFileName','char')  RTIBlockParaDefault=struct('VarName','Var1','DataType','Single','SampleTime',-1,'TLCFileName','rtiusbflightrecwrite')
      settings: SourceProductName=dSPACE RTI USB Flight Rec Blockset
  USB_FLIGHT_REC_s5t4 : rtiusbflightreclib/USB_FLIGHT_REC_BL1  VarName=s5t4  DataType=Single  SampleTime=-1  TLCFileName=rtiusbflightrecwrite  Reserved1=[]  Reserved2=[]  Reserved3=[]  Reserved4=[]  DSProperties=struct('RTI',struct('Version',uint32(3),'BlockType',struct('isSLSource',uint8(0),'isSLSink',uint8(1),'isHWSource',uint8(0),'isHWSink',uint8(0),'isSetup',uint8(0),'isInline',uint8(1),'isNonInline',uint8(0),'isInterrupt',uint8(0),'isChannelwise',uint8(0)),'IOBoardType',{{'DSUSB','FLIGHTREC'}},'UnitType','FLIGHTREC','Identifier','WRITE','DialogType','SL','BlockSet','RTIUSBFLIGHTREC','SlaveProcessor','NONE'))  RTIBlockInterface=struct('InputPortsActive',1,'InputPortsWidth',int32(1),'InputPortsDataType',{{'SS_SINGLE'}},'BlockDisplay',{{['Write to\nUSB Flight Recorder'],'center'}},'IconTransparency','off','InitLevel',3,'BlockName',struct('Token',{{'USB_FLIGHT_REC_BL1'}}),'MaskDescription',['Write input to the Flight Recorder. Recorded data can be referenced by the specified variable.'],'SampleTime',{{-1}})  RTIBlockParameters=struct('VarName',{{'s5t4','OFF',[]}},'DataType',{{'Single','OFF',[]}},'SampleTime',{{-1,'OFF',[]}},'TLCFileName',{{'rtiusbflightrecwrite','OFF',[]}})  RTISFcnParameters=struct('VarName','char','DataType','char','SampleTime','double','TLCFileName','char')  RTIBlockParaDefault=struct('VarName','Var1','DataType','Single','SampleTime',-1,'TLCFileName','rtiusbflightrecwrite')
      settings: SourceProductName=dSPACE RTI USB Flight Rec Blockset
  s5c{1..12} (12 alike) : Gain  Gain=0.0015
  s5t1 : MATLAB Function  TreatAsAtomicUnit=on
  s5t2 : MATLAB Function  TreatAsAtomicUnit=on
  s5t3 : MATLAB Function  TreatAsAtomicUnit=on
  s5t4 : MATLAB Function  TreatAsAtomicUnit=on
  s5temp{1..4} (4 alike) : Gain  Gain=0.0015
  CAN Error s5 : Outport
  Max Voltage s5 : Outport  Port=2
  Min Voltage s5 : Outport  Port=3
  Voltage Sum s5 : Outport  Port=4
  Max Temperature s5 : Outport  Port=5
  Min Temperature s5 : Outport  Port=6
  wires:
  Data Type Conversion6/1 -> Add2/1
  Gain_s5c10/1 -> Data Type Conversion19/1
  BMS_218/6 -> 218_Error/1
  Gain_s5c11/1 -> Data Type Conversion16/1
  218_Error/1 -> CAN_s5_Error/1
  Edge Detector3/1 -> Data Type Conversion6/1
  BMS_CAN_218_Counter/1 -> Add2/2
  Add2/1 -> BMS_CAN_218_Counter/1
  Gain_s5c9/1 -> Data Type Conversion18/1
  Gain_s5c12/1 -> Data Type Conversion17/1
  BMS_218/5 -> Edge Detector3/1
  s5c7/1 -> Add_Voltage_s5q2/2, Min_Voltage_s5q2/2, Max_Voltage_s5q2/2, Gain_s5c7/1
  BMS_217/6 -> 217_Error/1
  Edge Detector2/1 -> Data Type Conversion5/1
  s5c5/1 -> Add_Voltage_s5q2/4, Min_Voltage_s5q2/4, Max_Voltage_s5q2/4, Gain_s5c5/1
  217_Error/1 -> CAN_s5_Error/2
  Gain_s5c5/1 -> Data Type Conversion10/1
  s5c6/1 -> Add_Voltage_s5q2/3, Min_Voltage_s5q2/3, Max_Voltage_s5q2/3, Gain_s5c6/1
  Gain_s5c6/1 -> Data Type Conversion11/1
  s5c8/1 -> Add_Voltage_s5q2/1, Min_Voltage_s5q2/1, Max_Voltage_s5q2/1, Gain_s5c8/1
  Data Type Conversion5/1 -> Add1/1
  Add1/1 -> BMS_CAN_217_Counter/1
  Gain_s5c8/1 -> Data Type Conversion9/1
  BMS_217/5 -> Edge Detector2/1
  Gain_s5c7/1 -> Data Type Conversion8/1
  BMS_CAN_217_Counter/1 -> Add1/2
  s5c2/1 -> Add_Voltage_s5q1/3, Min_Voltage_s5q1/3, Max_Voltage_s5q1/3, Gain_s5c2/1
  Gain_s5c2/1 -> Data Type Conversion15/1
  216_Error/1 -> CAN_s5_Error/3
  s5c1/1 -> Add_Voltage_s5q1/4, Min_Voltage_s5q1/4, Max_Voltage_s5q1/4, Gain_s5c1/1
  Max_Voltage_s5q3/1 -> Max_Voltage_s5/1
  Gain_s5c1/1 -> Data Type Conversion14/1
  s5c4/1 -> Add_Voltage_s5q1/1, Min_Voltage_s5q1/1, Max_Voltage_s5q1/1, Gain_s5c4/1
  Gain_s5c4/1 -> Data Type Conversion13/1
  Gain_s5c3/1 -> Data Type Conversion12/1
  s5c3/1 -> Add_Voltage_s5q1/2, Min_Voltage_s5q1/2, Max_Voltage_s5q1/2, Gain_s5c3/1
  Add_Voltage_s5q2/1 -> Add_Voltage_s5/2
  Min_Voltage_s5q1/1 -> Min_Voltage_s5/3
  Max_Voltage_s5q2/1 -> Max_Voltage_s5/2
  BMS_216/6 -> 216_Error/1
  BMS_CAN_216_Counter/1 -> Add4/2
  Edge Detector1/1 -> Data Type Conversion4/1
  Add4/1 -> BMS_CAN_216_Counter/1
  Data Type Conversion4/1 -> Add4/1
  BMS_216/5 -> Edge Detector1/1
  Min_Voltage_s5q2/1 -> Min_Voltage_s5/2
  Max_Voltage_s5q1/1 -> Max_Voltage_s5/3
  Add_Voltage_s5q1/1 -> Add_Voltage_s5/3
  Add_Voltage_s5q3/1 -> Add_Voltage_s5/1
  Max_Voltage_s5/1 -> Max Voltage s5/1
  CAN_s5_Error/1 -> CAN Error s5/1
  Min_Voltage_s5/1 -> Min Voltage s5/1
  Add_Voltage_s5/1 -> Voltage Sum s5/1
  Min_Voltage_s5q3/1 -> Min_Voltage_s5/1
  s5c10/1 -> Add_Voltage_s5q3/3, Min_Voltage_s5q3/3, Max_Voltage_s5q3/3, Gain_s5c10/1
  s5c9/1 -> Add_Voltage_s5q3/4, Min_Voltage_s5q3/4, Max_Voltage_s5q3/4, Gain_s5c9/1
  s5c11/1 -> Add_Voltage_s5q3/2, Min_Voltage_s5q3/2, Max_Voltage_s5q3/2, Gain_s5c11/1
  s5c12/1 -> Add_Voltage_s5q3/1, Min_Voltage_s5q3/1, Max_Voltage_s5q3/1, Gain_s5c12/1
  BMS_229/6 -> 229_Error/1
  BMS_CAN_229_Counter/1 -> Add3/2
  Add3/1 -> BMS_CAN_229_Counter/1
  Edge Detector4/1 -> Data Type Conversion1/1
  s5t3/1(y) -> Min_Temp_s5t/2, Max_Temp_s5t/2, Gain_s5t3/1
  s5t4/1(y) -> Min_Temp_s5t/1, Max_Temp_s5t/1, Gain_s5t4/1
  BMS_229/5 -> Edge Detector4/1
  s5t1/1(y) -> Min_Temp_s5t/4, Max_Temp_s5t/4, Gain_s5t1/1
  s5t2/1(y) -> Min_Temp_s5t/3, Max_Temp_s5t/3, Gain_s5t2/1
  Data Type Conversion1/1 -> Add3/1
  s5temp1/1 -> s5t1/1(x)
  s5temp2/1 -> s5t2/1(x)
  s5temp3/1 -> s5t3/1(x)
  s5temp4/1 -> s5t4/1(x)
  Gain_s5t1/1 -> USB_FLIGHT_REC_s5t1/1
  Gain_s5t4/1 -> USB_FLIGHT_REC_s5t4/1
  Gain_s5t3/1 -> USB_FLIGHT_REC_s5t3/1
  Gain_s5t2/1 -> USB_FLIGHT_REC_s5t2/1
  Min_Temp_s5t/1 -> Min Temperature s5/1
  Max_Temp_s5t/1 -> Max Temperature s5/1
  229_Error/1 -> CAN_s5_Error/4
  BMS_229/4 -> Data Type Conversion7/1  "s5t4"
  BMS_229/3 -> Data Type Conversion3/1  "s5t3"
  BMS_229/2 -> Data Type Conversion2/1  "s5t2"
  BMS_229/1 -> Data Type Conversion/1  "s5t1"
  BMS_216/4 -> s5c4/1  "s5c4"
  BMS_216/3 -> s5c3/1  "s5c3"
  BMS_216/2 -> s5c2/1  "s5c2"
  BMS_216/1 -> s5c1/1  "s5c1"
  BMS_218/1 -> s5c9/1  "s5c5"
  BMS_218/2 -> s5c10/1  "s5c6"
  BMS_218/3 -> s5c11/1  "s5c7"
  BMS_218/4 -> s5c12/1  "s5c8"
  BMS_217/4 -> s5c8/1  "s5c8"
  BMS_217/3 -> s5c7/1  "s5c7"
  BMS_217/2 -> s5c6/1  "s5c6"
  BMS_217/1 -> s5c5/1  "s5c5"
  Data Type Conversion3/1 -> s5temp3/1
  Data Type Conversion/1 -> s5temp1/1
  Data Type Conversion2/1 -> s5temp2/1
  Data Type Conversion7/1 -> s5temp4/1
  Data Type Conversion13/1 -> USB_FLIGHT_REC_s5c4/1
  Data Type Conversion12/1 -> USB_FLIGHT_REC_s5c3/1
  Data Type Conversion15/1 -> USB_FLIGHT_REC_s5c2/1
  Data Type Conversion14/1 -> USB_FLIGHT_REC_s5c1/1
  Data Type Conversion8/1 -> USB_FLIGHT_REC_s5c7/1
  Data Type Conversion11/1 -> USB_FLIGHT_REC_s5c6/1
  Data Type Conversion10/1 -> USB_FLIGHT_REC_s5c5/1
  Data Type Conversion9/1 -> USB_FLIGHT_REC_s5c8/1
  Data Type Conversion19/1 -> USB_FLIGHT_REC_s5c10/1
  Data Type Conversion17/1 -> USB_FLIGHT_REC_s5c12/1
  Data Type Conversion16/1 -> USB_FLIGHT_REC_s5c11/1
  Data Type Conversion18/1 -> USB_FLIGHT_REC_s5c9/1
